simulink model "loadedInverter"  (R2024a)
settings: Solver=ode113  StartTime=0  StopTime=5  FixedStep=1e-6  RelTol=1e-8
libraries: simulink x7, spsIGBTDiodeLib x6, spsThreePhaseSeriesRLCBranchLib x3, spsGroundLib x2, spsPermanentMagnetSynchronousMachineLib x2, spsDCVoltageSourceLib x1, spsThreePhaseVIMeasurementLib x1, sps_lib x1
settings Model: Creator=ammarabdulrasheed  LastModifiedBy=ammarabdulrasheed
settings DataIOCC: ReturnWorkspaceOutputs=off

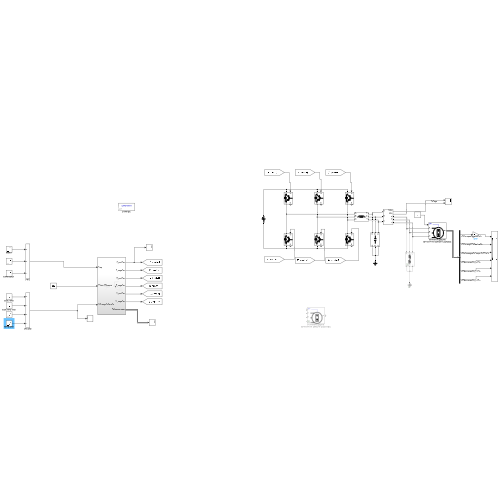
[thumbnail: Simulink's stored preview of the top-level diagram]
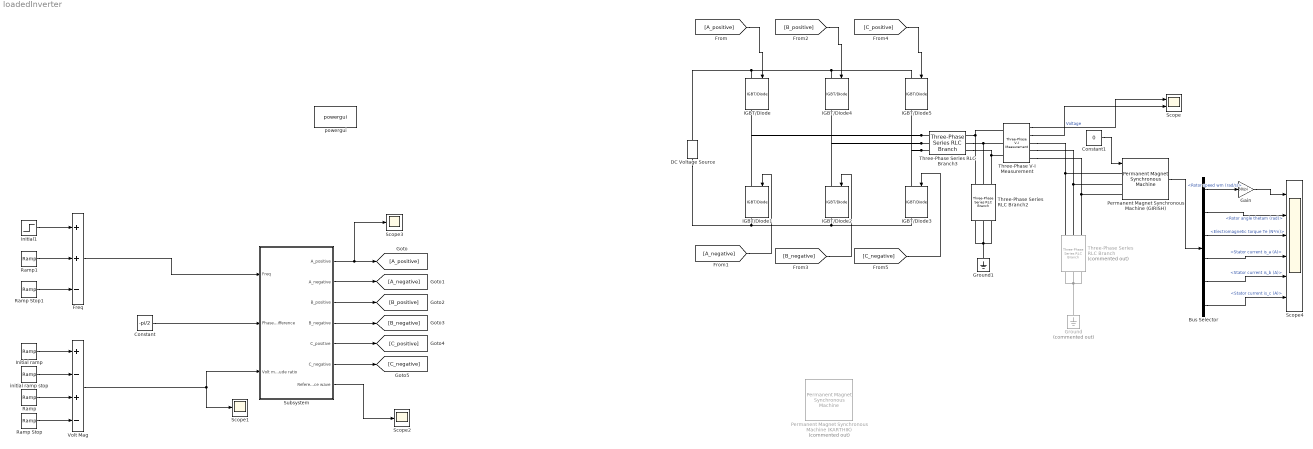
== system loadedInverter ==
  Bus Selector : BusSelector  OutputSignals=Rotor speed wm (rad/s),Rotor angle thetam (rad),Electromagnetic torque Te (N*m),Stator current is_a (A),Stator current is_b (A),Stator current is_c (A)
  Constant : Constant  Value=-pi/2
  Constant1 : Constant  Value=0
  DC Voltage Source : spsDCVoltageSourceLib/DC Voltage Source  Amplitude=400  Measurements=None
  Freq : Sum  Inputs=++-
  Gain : Gain  Gain=30/pi
  Ground : spsGroundLib/Ground  Commented=on  LConnTagsString=a
  Ground1 : spsGroundLib/Ground  LConnTagsString=a
  IGBT/Diode{,1..5} (6 alike) : spsIGBTDiodeLib/IGBT//Diode  Ron=1e-3  Rs=1e5  Cs=inf  Measurements=on
  Initial ramp : simulink/Sources/Ramp  slope=0.08  start=0  InitialOutput=0
  Initial1 : Step  Time=0  After=0  SampleTime=0
  Permanent Magnet Synchronous Machine (GIRISH) : spsPermanentMagnetSynchronousMachineLib/Permanent Magnet Synchronous Machine  NbPhases=3  FluxDistribution=Sinusoidal  RotorType=Salient-pole  MechanicalLoad=Torque Tm  PresetModel=No  ShowDetailedParameters=on  MeasurementBus=off  Resistance=1.93  Inductance=8.5e-3  dqInductances=[45.56e-3,79.57e-3]  La=92.19e-3  MachineConstant=Flux linkage established by magnets (V.s)  Flux=0.311  VoltageCst=112.8183  TorqueCst=0.933  Flat=120  Mechanical=[0.003 0.001 2 0]  PolePairs=4  InitialConditions=[0,0, 0,0]  InitialConditions5ph=[0 0 0 0 0 0]  RefAngle=90 degrees behind phase A axis (modified Park)  IterativeDiscreteModel=Trapezoidal non iterative  TsBlock=-1  TsPowergui=0
  Permanent Magnet Synchronous Machine (KARTHIK) : spsPermanentMagnetSynchronousMachineLib/Permanent Magnet Synchronous Machine  Commented=on  NbPhases=3  FluxDistribution=Sinusoidal  RotorType=Round  MechanicalLoad=Torque Tm  PresetModel=No  ShowDetailedParameters=on  MeasurementBus=off  Resistance=1.15  Inductance=8.5e-3  dqInductances=[45.56e-3,79.57e-3]  La=24.3e-3  MachineConstant=Flux linkage established by magnets (V.s)  Flux=0.9426  VoltageCst=341.9375  TorqueCst=2.8278  Flat=120  Mechanical=[0.0145 0.00029 2 0]  PolePairs=4  InitialConditions=[0,0, 0,0]  InitialConditions5ph=[0 0 0 0 0 0]  RefAngle=90 degrees behind phase A axis (modified Park)  IterativeDiscreteModel=Trapezoidal non iterative  TsBlock=-1  TsPowergui=0
  Ramp : simulink/Sources/Ramp  slope=(50/3)*(1/50)  start=1 + 0.06  InitialOutput=0
  Ramp Stop : simulink/Sources/Ramp  slope=(50/3)*(1/50)  start=3  InitialOutput=0
  Ramp Stop1 : simulink/Sources/Ramp  slope=50/3  start=3  InitialOutput=0
  Ramp1 : simulink/Sources/Ramp  slope=50/3  start=1  InitialOutput=0
  Scope : Scope  NumInputPorts=2
  Scope1 : Scope
  Scope2 : Scope
  Scope3 : Scope
  Scope4 : Scope  NumInputPorts=6
  Subsystem : Subsystem
  Three-Phase Series RLC Branch : spsThreePhaseSeriesRLCBranchLib/Three-Phase Series RLC Branch  Commented=on  LConnTagsString=A|B|C  RConnTagsString=A|B|C  BranchType=RL  Resistance=2  Inductance=90e-3  Capacitance=1e-6  Measurements=None
  Three-Phase Series RLC Branch2 : spsThreePhaseSeriesRLCBranchLib/Three-Phase Series RLC Branch  LConnTagsString=A|B|C  RConnTagsString=A|B|C  BranchType=C  Resistance=1e-6  Inductance=1e-3  Capacitance=250e-6  Measurements=None
  Three-Phase Series RLC Branch3 : spsThreePhaseSeriesRLCBranchLib/Three-Phase Series RLC Branch  LConnTagsString=A|B|C  RConnTagsString=A|B|C  BranchType=L  Resistance=1  Inductance=1e-3  Capacitance=1e-6  Measurements=None
  Three-Phase V-I Measurement : spsThreePhaseVIMeasurementLib/Three-Phase V-I Measurement  VoltageMeasurement=phase-to-ground  SetLabelV=off  LabelV=Vabc  Vpu=off  VpuLL=off  CurrentMeasurement=yes  SetLabelI=off  LabelI=Iabc  Ipu=off  Pbase=100e6  Vbase=500e3  OutputType=Complex  PhasorSimulation=off  PSBequivalent=0
  Volt Mag : Sum  Inputs=+-+-
  initial ramp stop : simulink/Sources/Ramp  slope=0.08  start=0.25  InitialOutput=0
  powergui : sps_lib/powergui  Priority=1  SimulationMode=Continuous  SampleTime=50e-6  frequency=60  Iterations=50  frequencyindice=0  Pbase=100e6  ErrMax=1e-4  UnitsV=kV  UnitsW=MW  buscounter=0  FunctionMessages=off  echomessages=off  EnableUseOfTLC=off  CurrentSourceSwitches=off  DisableSnubberDevices=off  DisableRonSwitches=off  DisableVfSwitches=off  DisplayEquations=off  AutomaticDiscreteSolvers=off  SolverType=Tustin/Backward Euler (TBE)  Interpol=off  ExternalGateDelay=off  methode=off  Ts=100  x0status=blocks  SPID=on  SwTol=0  HookPort=off  NonlinearTolerance=1e-4  nMaxIteration=100  ContinueOnMaxIteration=off  RestoreLinks=warning  ResistiveCurrentMeasurement=off  Frange=[0:2:500]  Ylog=off  Xlog=on  ShowGrid=off  save=off  variable=ZData  structure=0  ZoomFFT=off  StartTime=0.0  cycles=1  DisplayStyle=1  fundamental=60  FreqAxis=off  MaxFrequency=1000  frequencyindicesteady=1  RmsSteady=1  display=off
  wires:
  Initial ramp/1 -> Volt Mag/1
  Ramp Stop/1 -> Volt Mag/4
  initial ramp stop/1 -> Volt Mag/2
  Ramp/1 -> Volt Mag/3
  Initial1/1 -> Freq/1
  Volt Mag/1 -> Scope1/1, Subsystem/3(Volt magnitude ratio)
  Freq/1 -> Subsystem/1(Freq)
  Constant/1 -> Subsystem/2(Phase Difference)
  Subsystem/1(A_positive) -> Scope3/1, [A_positive]
  Subsystem/2(A_negative) -> [A_negative]
  Subsystem/3(B_positive) -> [B_positive]
  Subsystem/4(B_negative) -> [B_negative]
  Subsystem/5(C_positive) -> [C_positive]
  Subsystem/6(C_negative) -> [C_negative]
  [A_positive] -> IGBT/Diode/1
  [B_positive] -> IGBT/Diode4/1
  [C_positive] -> IGBT/Diode5/1
  [C_negative] -> IGBT/Diode3/1
  [B_negative] -> IGBT/Diode2/1
  [A_negative] -> IGBT/Diode1/1
  Subsystem/7(Reference wave) -> Scope2/1
  Three-Phase V-I Measurement/1 -> Scope/1  "Voltage"
  Three-Phase V-I Measurement/2 -> Scope/2
  Constant1/1 -> Permanent Magnet Synchronous Machine (GIRISH)/1
  Permanent Magnet Synchronous Machine (GIRISH)/1 -> Bus Selector/1
  Bus Selector/2 -> Scope4/2  "<Rotor angle thetam (rad)>"
  Bus Selector/4 -> Scope4/4  "<Stator current is_a (A)>"
  Bus Selector/5 -> Scope4/5  "<Stator current is_b (A)>"
  Bus Selector/6 -> Scope4/6  "<Stator current is_c (A)>"
  Ramp1/1 -> Freq/2
  Ramp Stop1/1 -> Freq/3
  Bus Selector/3 -> Scope4/3  "<Electromagnetic torque Te (N*m)>"
  Bus Selector/1 -> Gain/1  "<Rotor speed wm (rad/s)>"
  Gain/1 -> Scope4/1
  connections:
  DC Voltage Source/RConn1 -- IGBT/Diode5/LConn1 -- IGBT/Diode4/LConn1 -- IGBT/Diode/LConn1
  DC Voltage Source/LConn1 -- IGBT/Diode3/RConn1 -- IGBT/Diode2/RConn1 -- IGBT/Diode1/RConn1
  Three-Phase Series RLC Branch2/LConn1 -- Three-Phase Series RLC Branch3/RConn1 -- Three-Phase V-I Measurement/LConn1
  Three-Phase Series RLC Branch3/LConn2 -- IGBT/Diode4/RConn1 -- IGBT/Diode2/LConn1
  Three-Phase Series RLC Branch3/LConn3 -- IGBT/Diode5/RConn1 -- IGBT/Diode3/LConn1
  Three-Phase V-I Measurement/RConn1 -- Three-Phase Series RLC Branch/LConn1 -- Permanent Magnet Synchronous Machine (GIRISH)/LConn1
  Three-Phase V-I Measurement/RConn2 -- Permanent Magnet Synchronous Machine (GIRISH)/LConn2 -- Three-Phase Series RLC Branch/LConn2
  Three-Phase V-I Measurement/RConn3 -- Permanent Magnet Synchronous Machine (GIRISH)/LConn3 -- Three-Phase Series RLC Branch/LConn3
  Ground/LConn1 -- Three-Phase Series RLC Branch/RConn1 -- Three-Phase Series RLC Branch/RConn3 -- Three-Phase Series RLC Branch/RConn2
  Ground1/LConn1 -- Three-Phase Series RLC Branch2/RConn3 -- Three-Phase Series RLC Branch2/RConn1 -- Three-Phase Series RLC Branch2/RConn2
  Three-Phase Series RLC Branch3/LConn1 -- IGBT/Diode1/LConn1 -- IGBT/Diode/RConn1
  Three-Phase Series RLC Branch2/LConn2 -- Three-Phase V-I Measurement/LConn2 -- Three-Phase Series RLC Branch3/RConn2
  Three-Phase Series RLC Branch2/LConn3 -- Three-Phase Series RLC Branch3/RConn3 -- Three-Phase V-I Measurement/LConn3

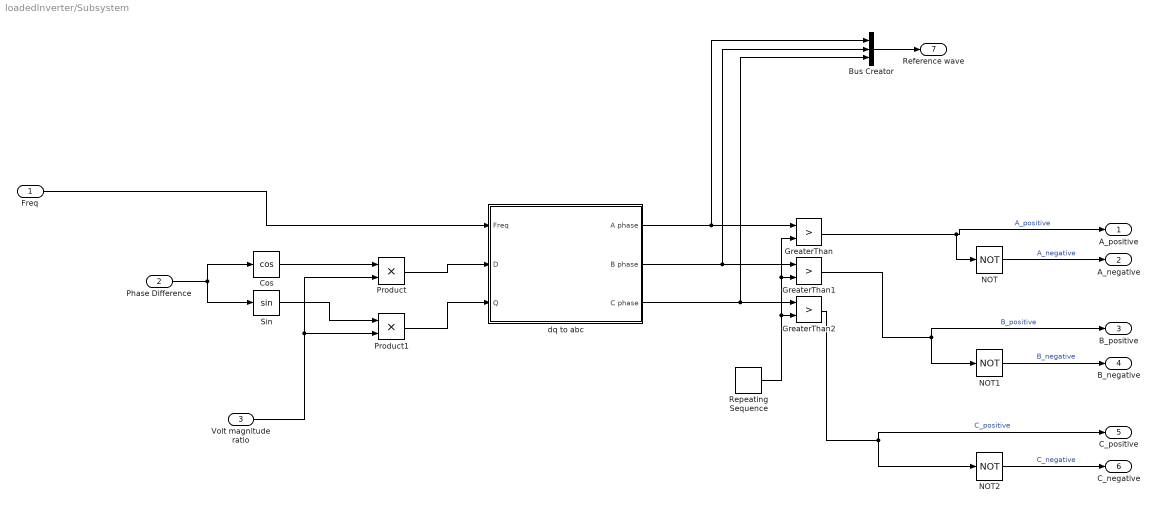
== system loadedInverter/Subsystem ==
  Freq : Inport
  Phase Difference : Inport  Port=2
  Volt magnitude ratio : Inport  Port=3
  Bus Creator : BusCreator  Inputs=3
  Cos : Trigonometry  Operator=cos
  GreaterThan : RelationalOperator  Operator=>  OutDataTypeStr=boolean  RndMeth=Simplest  InputSameDT=off
  GreaterThan1 : RelationalOperator  Operator=>  OutDataTypeStr=boolean  RndMeth=Simplest  InputSameDT=off
  GreaterThan2 : RelationalOperator  Operator=>  OutDataTypeStr=boolean  RndMeth=Simplest  InputSameDT=off
  NOT : Logic  Operator=NOT  IconShape=distinctive  AllPortsSameDT=off  OutDataTypeStr=boolean
  NOT1 : Logic  Operator=NOT  IconShape=distinctive  AllPortsSameDT=off  OutDataTypeStr=boolean
  NOT2 : Logic  Operator=NOT  IconShape=distinctive  AllPortsSameDT=off  OutDataTypeStr=boolean
  Product : Product
  Product1 : Product
  Repeating Sequence : simulink/Sources/Repeating Sequence  rep_seq_t=[0 1 2 3 4]*(1/5)*0.5e-3  rep_seq_y=[0 1 0 -1 0]
  Sin : Trigonometry
  dq to abc : Subsystem
  A_positive : Outport
  A_negative : Outport  Port=2
  B_positive : Outport  Port=3
  B_negative : Outport  Port=4
  C_positive : Outport  Port=5
  C_negative : Outport  Port=6
  Reference wave : Outport  Port=7
  wires:
  NOT2/1 -> C_negative/1  "C_negative"
  Product1/1 -> dq to abc/3(Q)
  Phase Difference/1 -> Sin/1, Cos/1
  NOT1/1 -> B_negative/1  "B_negative"
  Repeating Sequence/1 -> GreaterThan/2, GreaterThan1/2, GreaterThan2/2
  Sin/1 -> Product1/1
  Volt magnitude ratio/1 -> Product1/2, Product/2
  Cos/1 -> Product/1
  NOT/1 -> A_negative/1  "A_negative"
  GreaterThan/1 -> A_positive/1, NOT/1  "A_positive"
  GreaterThan1/1 -> B_positive/1, NOT1/1  "B_positive"
  GreaterThan2/1 -> C_positive/1, NOT2/1  "C_positive"
  Product/1 -> dq to abc/2(D)
  dq to abc/2(B phase) -> Bus Creator/2, GreaterThan1/1
  dq to abc/3(C phase) -> Bus Creator/3, GreaterThan2/1
  Freq/1 -> dq to abc/1(Freq)
  dq to abc/1(A phase) -> Bus Creator/1, GreaterThan/1
  Bus Creator/1 -> Reference wave/1

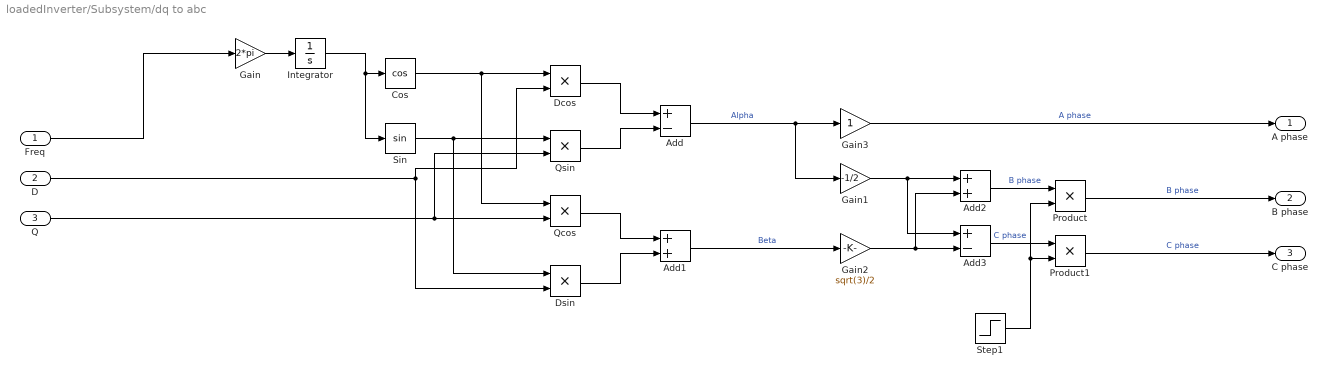
== system loadedInverter/Subsystem/dq to abc ==
  Freq : Inport
  D : Inport  Port=2
  Q : Inport  Port=3
  Add : Sum  Inputs=+-
  Add1 : Sum
  Add2 : Sum
  Add3 : Sum  Inputs=+-
  Cos : Trigonometry  Operator=cos
  Dcos : Product
  Dsin : Product
  Gain : Gain  Gain=2*pi
  Gain1 : Gain  Gain=-1/2
  Gain2 : Gain  Gain=sqrt(3)/2
  Gain3 : Gain
  Integrator : Integrator
  Product : Product
  Product1 : Product
  Qcos : Product
  Qsin : Product
  Sin : Trigonometry
  Step1 : Step  Time=0  SampleTime=0
  A phase : Outport
  B phase : Outport  Port=2
  C phase : Outport  Port=3
  wires:
  Product/1 -> B phase/1  "B phase"
  Add1/1 -> Gain2/1  "Beta"
  Product1/1 -> C phase/1  "C phase"
  D/1 -> Dsin/2, Dcos/2
  Dsin/1 -> Add1/2
  Freq/1 -> Gain/1
  Step1/1 -> Product1/2, Product/2
  Q/1 -> Qcos/2, Qsin/2
  Dcos/1 -> Add/1
  Gain/1 -> Integrator/1
  Gain3/1 -> A phase/1  "A phase"
  Cos/1 -> Qcos/1, Dcos/1
  Add2/1 -> Product/1  "B phase"
  Gain2/1 -> Add3/2, Add2/2
  Integrator/1 -> Sin/1, Cos/1
  Add3/1 -> Product1/1  "C phase"
  Sin/1 -> Dsin/1, Qsin/1
  Gain1/1 -> Add3/1, Add2/1
  Qsin/1 -> Add/2
  Qcos/1 -> Add1/1
  Add/1 -> Gain1/1, Gain3/1  "Alpha"
